simulink model "sim_sfrd"  (R2013a)
settings: Solver=ode45  StartTime=0.0  StopTime=25  RelTol=1e-3
settings Model: Creator=Aleksandr  LastModifiedBy=Aleksandr

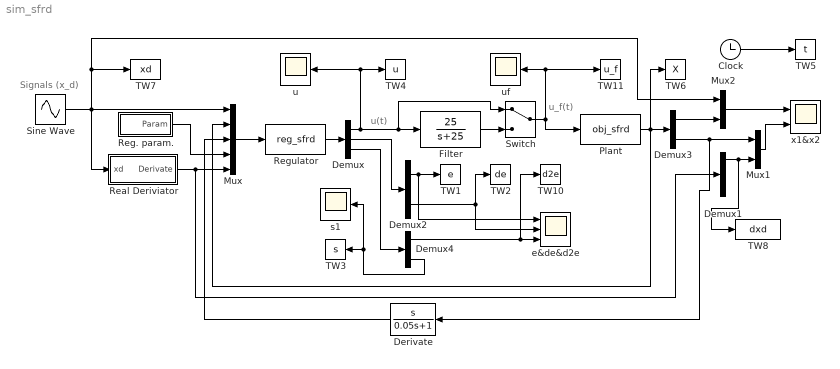
== system sim_sfrd ==
  note: u_f(t)
  note: u(t)
  note: Signals (x_d)
  Clock : Clock
      settings: Decimation=15
  Demux : Demux  Outputs=3
  Demux1 : Demux  Outputs=3
  Demux2 : Demux  Outputs=2
  Demux3 : Demux  Outputs=2
  Demux4 : Demux  Outputs=2
  Derivate : TransferFcn  Numerator=[1 0]  Denominator=[0.05 1]
  Filter : TransferFcn  Numerator=[0 25]  Denominator=[1 25]
  Mux : Mux  Inputs=5
  Mux1 : Mux  Inputs=2
  Mux2 : Mux  Inputs=2
  Plant : S-Function  FunctionName=obj_sfrd  EnableBusSupport=off
  Real Deriviator : Subsystem
  Reg. param. : Subsystem
  Regulator : S-Function  FunctionName=reg_sfrd  EnableBusSupport=off
  Sine Wave : Sin  SampleTime=0
  Switch : ManualSwitch
  TW1 : ToWorkspace  VariableName=e  SampleTime=-1
  TW10 : ToWorkspace  VariableName=d2e  SampleTime=-1
  TW11 : ToWorkspace  VariableName=u_f  SampleTime=-1
  TW2 : ToWorkspace  VariableName=de  SampleTime=-1
  TW3 : ToWorkspace  VariableName=s  SampleTime=-1
  TW4 : ToWorkspace  VariableName=u  SampleTime=-1
  TW5 : ToWorkspace  VariableName=t  SampleTime=-1
  TW6 : ToWorkspace  VariableName=X  SampleTime=-1
  TW7 : ToWorkspace  VariableName=xd  SampleTime=-1
  TW8 : ToWorkspace  VariableName=dxd  SampleTime=-1
  e&de&d2e : Scope  NumInputPorts=3
      settings: TimeRange=20  YMin=-5~-5~-5  YMax=5~5~5
  s1 : Scope
      settings: SaveName=ScopeData4
  u : Scope
      settings: SaveName=ScopeData3
  uf : Scope
      settings: SaveName=ScopeData5
  x1&x2 : Scope  NumInputPorts=2
      settings: TimeRange=20  YMin=-5~-5  YMax=5~5  SaveName=ScopeData2
  wires:
  Clock/1 -> TW5/1
  Regulator/1 -> Demux/1
  Demux/1 -> Switch/1, Filter/1, TW4/1, u/1
  Demux2/1 -> e&de&d2e/1, TW1/1
  Plant/1 -> TW6/1, Demux3/1, Mux/2
  Mux/1 -> Regulator/1
  Sine Wave/1 -> TW7/1, Mux2/1, Real Deriviator/1(xd), Mux/1
  Reg. param./1("Param ") -> Mux/4
  Real Deriviator/1(Derivate) -> Demux1/1, Mux/5
  Demux3/1 -> Mux2/2
  Mux2/1 -> x1&x2/1
  Demux1/1 -> TW8/1, Mux1/2
  Mux1/1 -> x1&x2/2
  Demux/2 -> Demux2/1
  Demux2/2 -> e&de&d2e/2, TW2/1
  Demux4/1 -> e&de&d2e/3, TW10/1
  Demux/3 -> Demux4/1
  Demux4/2 -> s1/1, TW3/1
  Switch/1 -> Plant/1, uf/1, TW11/1
  Filter/1 -> Switch/2
  Derivate/1 -> Mux/3
  Demux3/2 -> Derivate/1, Mux1/1

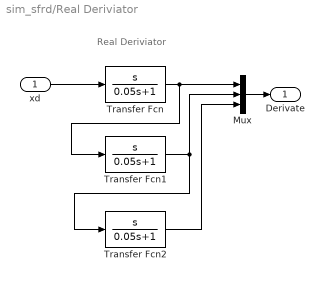
== system sim_sfrd/Real Deriviator ==
  note: Real Deriviator
  xd : Inport
  Mux : Mux  Inputs=3
  Transfer Fcn : TransferFcn  Numerator=[1 0]  Denominator=[0.05 1]
  Transfer Fcn1 : TransferFcn  Numerator=[1 0]  Denominator=[0.05 1]
  Transfer Fcn2 : TransferFcn  Numerator=[1 0]  Denominator=[0.05 1]
  Derivate : Outport
  wires:
  Transfer Fcn/1 -> Mux/1, Transfer Fcn1/1
  xd/1 -> Transfer Fcn/1
  Transfer Fcn1/1 -> Mux/2, Transfer Fcn2/1
  Transfer Fcn2/1 -> Mux/3
  Mux/1 -> Derivate/1

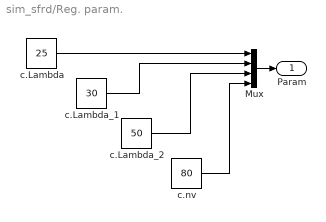
== system sim_sfrd/Reg. param. ==
  Mux : Mux
  c.Lambda : Constant  Value=25
  c.Lambda_1 : Constant  Value=30
  c.Lambda_2 : Constant  Value=50
  c.nv : Constant  Value=80
  "Param " : Outport
  wires:
  c.Lambda/1 -> Mux/1
  c.Lambda_1/1 -> Mux/2
  c.Lambda_2/1 -> Mux/3
  c.nv/1 -> Mux/4
  Mux/1 -> "Param "/1
